simulink model "zynqRadioHWSWLTEDetectorAD9361AD9364SL"  (R2016a)
settings: Solver=FixedStepDiscrete  SolverMode=SingleTasking  StartTime=0.0  StopTime=inf  RelTol=1e-3
InitFcn:
  | % Load LTE detector initialization parameters
  | simParams = hdlcoder_lteofdm_modDetectref_init;
  | simParams = hdlcoder_lteofdm_modDetecthdl_init(simParams);
  | 
  | % Modify PSS detection threshold gain for modified
  | % front-end filter
  | simParams.thresholdGain = 16;
  | 
  | % Load LTE TX waveforms
  | load('zynqRadioLTETransmitData');
libraries: simulink x26, hdlsllib x18, dspsigops x3, dspxfrm3 x1, dspmlti4 x1, dspmathops x1, dspsrcs4 x1
(part 2 of 2)

== system zynqRadioHWSWLTEDetectorAD9361AD9364SL/HDL_LTE/PSS_Detection/Cross_Correlation/Magnitude_Squared_0 ==
  dataIn : Inport
  Add : Sum  OutDataTypeStr=Inherit: Same as accumulator
  Complex to Real-Imag : ComplexToRealImag
  Delay1 : Delay  InitialCondition=0
  Delay2 : Delay  InitialCondition=0
  Delay3 : Delay  DelayLength=1  InitialCondition=0
  Delay4 : Delay  InitialCondition=0
  Product4 : Product
  Product5 : Product
  Magnitude^2 : Outport
  wires:
  Delay4/1 -> Magnitude^2/1
  Delay2/1 -> Add/2
  Delay1/1 -> Add/1
  Delay3/1 -> Complex to Real-Imag/1
  dataIn/1 -> Delay3/1
  Product4/1 -> Delay1/1
  Complex to Real-Imag/2 -> Product5/1, Product5/2
  Complex to Real-Imag/1 -> Product4/1, Product4/2
  Add/1 -> Delay4/1
  Product5/1 -> Delay2/1

== system zynqRadioHWSWLTEDetectorAD9361AD9364SL/HDL_LTE/PSS_Detection/Cross_Correlation/Magnitude_Squared_1 ==
  dataIn : Inport
  Add : Sum  OutDataTypeStr=Inherit: Same as accumulator
  Complex to Real-Imag : ComplexToRealImag
  Delay1 : Delay  InitialCondition=0
  Delay2 : Delay  InitialCondition=0
  Delay3 : Delay  DelayLength=1  InitialCondition=0
  Delay4 : Delay  InitialCondition=0
  Product4 : Product
  Product5 : Product
  Magnitude^2 : Outport
  wires:
  Delay4/1 -> Magnitude^2/1
  Delay2/1 -> Add/2
  Delay1/1 -> Add/1
  Delay3/1 -> Complex to Real-Imag/1
  dataIn/1 -> Delay3/1
  Product4/1 -> Delay1/1
  Complex to Real-Imag/2 -> Product5/1, Product5/2
  Complex to Real-Imag/1 -> Product4/1, Product4/2
  Add/1 -> Delay4/1
  Product5/1 -> Delay2/1

== system zynqRadioHWSWLTEDetectorAD9361AD9364SL/HDL_LTE/PSS_Detection/Cross_Correlation/Magnitude_Squared_2 ==
  dataIn : Inport
  Add : Sum  OutDataTypeStr=Inherit: Same as accumulator
  Complex to Real-Imag : ComplexToRealImag
  Delay1 : Delay  InitialCondition=0
  Delay2 : Delay  InitialCondition=0
  Delay3 : Delay  DelayLength=1  InitialCondition=0
  Delay4 : Delay  InitialCondition=0
  Product4 : Product
  Product5 : Product
  Magnitude^2 : Outport
  wires:
  Delay4/1 -> Magnitude^2/1
  Delay2/1 -> Add/2
  Delay1/1 -> Add/1
  Delay3/1 -> Complex to Real-Imag/1
  dataIn/1 -> Delay3/1
  Product4/1 -> Delay1/1
  Complex to Real-Imag/2 -> Product5/1, Product5/2
  Complex to Real-Imag/1 -> Product4/1, Product4/2
  Add/1 -> Delay4/1
  Product5/1 -> Delay2/1

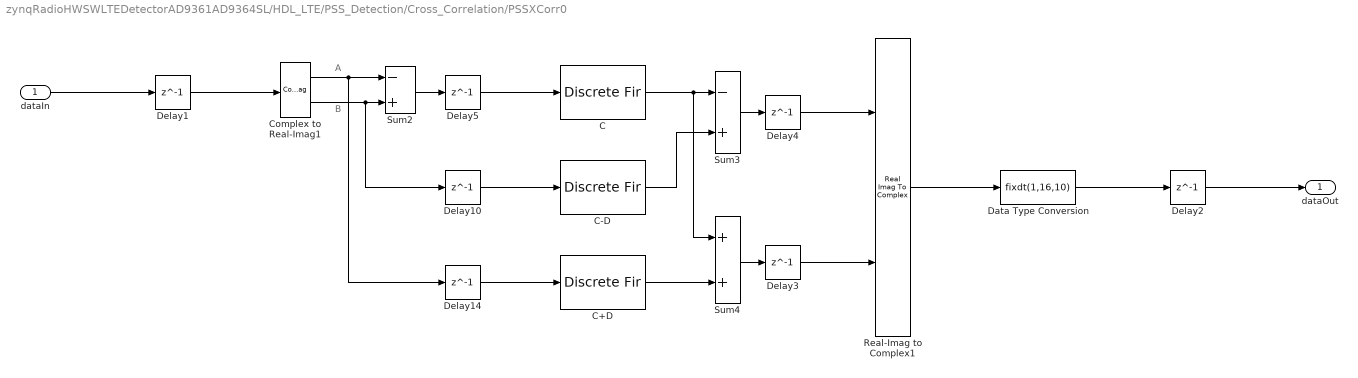
== system zynqRadioHWSWLTEDetectorAD9361AD9364SL/HDL_LTE/PSS_Detection/Cross_Correlation/PSSXCorr0 ==
  note: B
  note: A
  dataIn : Inport
  C : DiscreteFir  Coefficients=real(simParams.PSS(:,PSSIdx+1)')  CoefDataTypeStr=fixdt(1,18)
  C+D : DiscreteFir  Coefficients=real(simParams.PSS(:,PSSIdx+1)') + imag(simParams.PSS(:,PSSIdx+1)')  CoefDataTypeStr=fixdt(1,18)
  C-D : DiscreteFir  Coefficients=real(simParams.PSS(:,PSSIdx+1)') - imag(simParams.PSS(:,PSSIdx+1)')  CoefDataTypeStr=fixdt(1,18)
  Complex to Real-Imag1 : ComplexToRealImag
  Data Type Conversion : DataTypeConversion  OutDataTypeStr=fixdt(1,16,10)  RndMeth=Round
  Delay{1..5,10,14} (7 alike) : Delay  DelayLength=1  InitialCondition=0
  Real-Imag to Complex1 : RealImagToComplex
  Sum2 : Sum  Inputs=-+
  Sum3 : Sum  Inputs=-+
  Sum4 : Sum
  dataOut : Outport
  wires:
  dataIn/1 -> Delay1/1
  Real-Imag to Complex1/1 -> Data Type Conversion/1
  Sum2/1 -> Delay5/1
  Complex to Real-Imag1/1 -> Delay14/1, Sum2/1
  Complex to Real-Imag1/2 -> Delay10/1, Sum2/2
  C/1 -> Sum4/1, Sum3/1
  C-D/1 -> Sum3/2
  C+D/1 -> Sum4/2
  Sum3/1 -> Delay4/1
  Sum4/1 -> Delay3/1
  Delay1/1 -> Complex to Real-Imag1/1
  Delay2/1 -> dataOut/1
  Delay3/1 -> Real-Imag to Complex1/2
  Delay4/1 -> Real-Imag to Complex1/1
  Delay5/1 -> C/1
  Delay10/1 -> C-D/1
  Delay14/1 -> C+D/1
  Data Type Conversion/1 -> Delay2/1

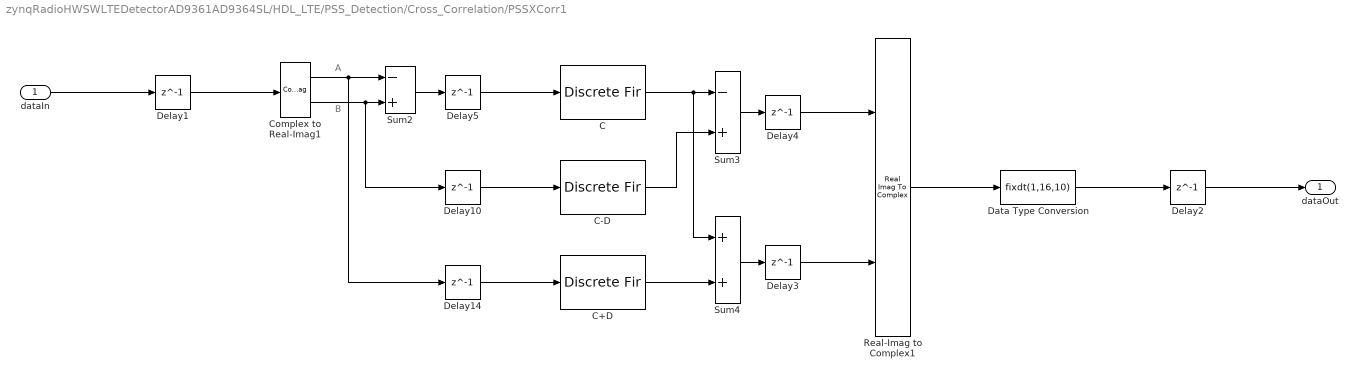
== system zynqRadioHWSWLTEDetectorAD9361AD9364SL/HDL_LTE/PSS_Detection/Cross_Correlation/PSSXCorr1 ==
  note: B
  note: A
  dataIn : Inport
  C : DiscreteFir  Coefficients=real(simParams.PSS(:,PSSIdx+1)')  CoefDataTypeStr=fixdt(1,18)
  C+D : DiscreteFir  Coefficients=real(simParams.PSS(:,PSSIdx+1)') + imag(simParams.PSS(:,PSSIdx+1)')  CoefDataTypeStr=fixdt(1,18)
  C-D : DiscreteFir  Coefficients=real(simParams.PSS(:,PSSIdx+1)') - imag(simParams.PSS(:,PSSIdx+1)')  CoefDataTypeStr=fixdt(1,18)
  Complex to Real-Imag1 : ComplexToRealImag
  Data Type Conversion : DataTypeConversion  OutDataTypeStr=fixdt(1,16,10)  RndMeth=Round
  Delay{1..5,10,14} (7 alike) : Delay  DelayLength=1  InitialCondition=0
  Real-Imag to Complex1 : RealImagToComplex
  Sum2 : Sum  Inputs=-+
  Sum3 : Sum  Inputs=-+
  Sum4 : Sum
  dataOut : Outport
  wires:
  dataIn/1 -> Delay1/1
  Real-Imag to Complex1/1 -> Data Type Conversion/1
  Sum2/1 -> Delay5/1
  Complex to Real-Imag1/1 -> Delay14/1, Sum2/1
  Complex to Real-Imag1/2 -> Delay10/1, Sum2/2
  C/1 -> Sum4/1, Sum3/1
  C-D/1 -> Sum3/2
  C+D/1 -> Sum4/2
  Sum3/1 -> Delay4/1
  Sum4/1 -> Delay3/1
  Delay1/1 -> Complex to Real-Imag1/1
  Delay2/1 -> dataOut/1
  Delay3/1 -> Real-Imag to Complex1/2
  Delay4/1 -> Real-Imag to Complex1/1
  Delay5/1 -> C/1
  Delay10/1 -> C-D/1
  Delay14/1 -> C+D/1
  Data Type Conversion/1 -> Delay2/1

== system zynqRadioHWSWLTEDetectorAD9361AD9364SL/HDL_LTE/PSS_Detection/Cross_Correlation/PSSXCorr2 ==
  note: B
  note: A
  dataIn : Inport
  C : DiscreteFir  Coefficients=real(simParams.PSS(:,PSSIdx+1)')  CoefDataTypeStr=fixdt(1,18)
  C+D : DiscreteFir  Coefficients=real(simParams.PSS(:,PSSIdx+1)') + imag(simParams.PSS(:,PSSIdx+1)')  CoefDataTypeStr=fixdt(1,18)
  C-D : DiscreteFir  Coefficients=real(simParams.PSS(:,PSSIdx+1)') - imag(simParams.PSS(:,PSSIdx+1)')  CoefDataTypeStr=fixdt(1,18)
  Complex to Real-Imag1 : ComplexToRealImag
  Data Type Conversion : DataTypeConversion  OutDataTypeStr=fixdt(1,16,10)  RndMeth=Round
  Delay{1..5,10,14} (7 alike) : Delay  DelayLength=1  InitialCondition=0
  Real-Imag to Complex1 : RealImagToComplex
  Sum2 : Sum  Inputs=-+
  Sum3 : Sum  Inputs=-+
  Sum4 : Sum
  dataOut : Outport
  wires:
  dataIn/1 -> Delay1/1
  Real-Imag to Complex1/1 -> Data Type Conversion/1
  Sum2/1 -> Delay5/1
  Complex to Real-Imag1/1 -> Delay14/1, Sum2/1
  Complex to Real-Imag1/2 -> Delay10/1, Sum2/2
  C/1 -> Sum4/1, Sum3/1
  C-D/1 -> Sum3/2
  C+D/1 -> Sum4/2
  Sum3/1 -> Delay4/1
  Sum4/1 -> Delay3/1
  Delay1/1 -> Complex to Real-Imag1/1
  Delay2/1 -> dataOut/1
  Delay3/1 -> Real-Imag to Complex1/2
  Delay4/1 -> Real-Imag to Complex1/1
  Delay5/1 -> C/1
  Delay10/1 -> C-D/1
  Delay14/1 -> C+D/1
  Data Type Conversion/1 -> Delay2/1

== system zynqRadioHWSWLTEDetectorAD9361AD9364SL/HDL_LTE/PSS_Detection/Peak_Detection/Local_Search_PSS0 ==
  note: Generate 10 sample enable signal
  Enb : Inport
  dataIn : Inport  Port=2
  indexIn : Inport  Port=3
  Add : Sum  AccumDataTypeStr=fixdt(0,15,0)
  Constant1 : Constant  Value=0  VectorParams1D=off  OutDataTypeStr=fixdt(0,22,20)  SampleTime=simParams.TsRx
  Constant2 : Constant  Value=11  VectorParams1D=off  OutDataTypeStr=fixdt(0,4,0)  SampleTime=simParams.TsRx
  Delay1 : Delay  DelayLength=11  InitialCondition=0
  Delay2 : Delay  DelayLength=1  InitialCondition=0
  Delay21 : Delay  DelayLength=1  InitialCondition=0  InputProcessing=Columns as channels (frame based)
  Delay3 : Delay  DelayLength=1  InitialCondition=0  InputProcessing=Columns as channels (frame based)
  HDL Counter : hdlsllib/HDL Operations/HDL Counter  CountType=Count limited  CountInit=1  CountStep=1  CountMax=11  CountFromType=Initial value  CountFrom=1  CountResetPort=off  CountLoadPort=off  CountEnbPort=on  CountDirPort=off  CountDataType=Unsigned  CountWordLen=4  CountFracLen=0  CountSampTime=1
  Logical Operator2 : Logic  Operator=OR  AllPortsSameDT=off  OutDataTypeStr=boolean
  Relational Operator1 : RelationalOperator  Operator=<  OutDataTypeStr=boolean
  Relational Operator2 : RelationalOperator  Operator=>  OutDataTypeStr=boolean
  Switch1 : Switch  Criteria=u2 ~= 0  Threshold=384
  maximum : Subsystem
  MaxIdx : Outport
  MaxVal : Outport  Port=2
  wires:
  Enb/1 -> Logical Operator2/1
  maximum/1(MaxVal) -> Delay21/1
  dataIn/1 -> Delay2/1
  maximum/2(MaxIdx) -> Relational Operator2/1, Add/1
  Add/1 -> Delay3/1
  Relational Operator2/1 -> Switch1/2
  indexIn/1 -> Delay1/1
  Constant1/1 -> Switch1/3, Relational Operator2/2
  Switch1/1 -> Add/2
  Delay1/1 -> Switch1/1
  Constant2/1 -> Relational Operator1/2
  Logical Operator2/1 -> HDL Counter/1
  Relational Operator1/1 -> maximum/2(Enb), Logical Operator2/2
  Delay2/1 -> maximum/1(dataIn)
  Delay21/1 -> MaxVal/1
  Delay3/1 -> MaxIdx/1
  HDL Counter/1 -> Relational Operator1/1

== system zynqRadioHWSWLTEDetectorAD9361AD9364SL/HDL_LTE/PSS_Detection/Peak_Detection/Local_Search_PSS1 ==
  note: Generate 10 sample enable signal
  Enb : Inport
  dataIn : Inport  Port=2
  indexIn : Inport  Port=3
  Add : Sum  AccumDataTypeStr=fixdt(0,15,0)
  Constant1 : Constant  Value=0  VectorParams1D=off  OutDataTypeStr=fixdt(0,22,20)  SampleTime=simParams.TsRx
  Constant2 : Constant  Value=11  VectorParams1D=off  OutDataTypeStr=fixdt(0,4,0)  SampleTime=simParams.TsRx
  Delay1 : Delay  DelayLength=11  InitialCondition=0
  Delay2 : Delay  DelayLength=1  InitialCondition=0
  Delay21 : Delay  DelayLength=1  InitialCondition=0  InputProcessing=Columns as channels (frame based)
  Delay3 : Delay  DelayLength=1  InitialCondition=0  InputProcessing=Columns as channels (frame based)
  HDL Counter : hdlsllib/HDL Operations/HDL Counter  CountType=Count limited  CountInit=1  CountStep=1  CountMax=11  CountFromType=Initial value  CountFrom=1  CountResetPort=off  CountLoadPort=off  CountEnbPort=on  CountDirPort=off  CountDataType=Unsigned  CountWordLen=4  CountFracLen=0  CountSampTime=1
  Logical Operator2 : Logic  Operator=OR  AllPortsSameDT=off  OutDataTypeStr=boolean
  Relational Operator1 : RelationalOperator  Operator=<  OutDataTypeStr=boolean
  Relational Operator2 : RelationalOperator  Operator=>  OutDataTypeStr=boolean
  Switch1 : Switch  Criteria=u2 ~= 0  Threshold=384
  maximum : Subsystem
  MaxIdx : Outport
  MaxVal : Outport  Port=2
  wires:
  HDL Counter/1 -> Relational Operator1/1
  Delay3/1 -> MaxIdx/1
  Delay21/1 -> MaxVal/1
  Delay2/1 -> maximum/1(dataIn)
  Relational Operator1/1 -> Logical Operator2/2, maximum/2(Enb)
  Logical Operator2/1 -> HDL Counter/1
  Constant2/1 -> Relational Operator1/2
  Delay1/1 -> Switch1/1
  Switch1/1 -> Add/2
  Constant1/1 -> Relational Operator2/2, Switch1/3
  indexIn/1 -> Delay1/1
  Relational Operator2/1 -> Switch1/2
  Add/1 -> Delay3/1
  maximum/2(MaxIdx) -> Add/1, Relational Operator2/1
  dataIn/1 -> Delay2/1
  maximum/1(MaxVal) -> Delay21/1
  Enb/1 -> Logical Operator2/1

== system zynqRadioHWSWLTEDetectorAD9361AD9364SL/HDL_LTE/PSS_Detection/Peak_Detection/Local_Search_PSS2 ==
  note: Generate 10 sample enable signal
  Enb : Inport
  dataIn : Inport  Port=2
  indexIn : Inport  Port=3
  Add : Sum  AccumDataTypeStr=fixdt(0,15,0)
  Constant1 : Constant  Value=0  VectorParams1D=off  OutDataTypeStr=fixdt(0,22,20)  SampleTime=simParams.TsRx
  Constant2 : Constant  Value=11  VectorParams1D=off  OutDataTypeStr=fixdt(0,4,0)  SampleTime=simParams.TsRx
  Delay1 : Delay  DelayLength=11  InitialCondition=0
  Delay2 : Delay  DelayLength=1  InitialCondition=0
  Delay21 : Delay  DelayLength=1  InitialCondition=0  InputProcessing=Columns as channels (frame based)
  Delay3 : Delay  DelayLength=1  InitialCondition=0  InputProcessing=Columns as channels (frame based)
  HDL Counter : hdlsllib/HDL Operations/HDL Counter  CountType=Count limited  CountInit=1  CountStep=1  CountMax=11  CountFromType=Initial value  CountFrom=1  CountResetPort=off  CountLoadPort=off  CountEnbPort=on  CountDirPort=off  CountDataType=Unsigned  CountWordLen=4  CountFracLen=0  CountSampTime=1
  Logical Operator2 : Logic  Operator=OR  AllPortsSameDT=off  OutDataTypeStr=boolean
  Relational Operator1 : RelationalOperator  Operator=<  OutDataTypeStr=boolean
  Relational Operator2 : RelationalOperator  Operator=>  OutDataTypeStr=boolean
  Switch1 : Switch  Criteria=u2 ~= 0  Threshold=384
  maximum : Subsystem
  MaxIdx : Outport
  MaxVal : Outport  Port=2
  wires:
  Enb/1 -> Logical Operator2/1
  maximum/1(MaxVal) -> Delay21/1
  dataIn/1 -> Delay2/1
  maximum/2(MaxIdx) -> Relational Operator2/1, Add/1
  Add/1 -> Delay3/1
  Relational Operator2/1 -> Switch1/2
  indexIn/1 -> Delay1/1
  Constant1/1 -> Switch1/3, Relational Operator2/2
  Switch1/1 -> Add/2
  Delay1/1 -> Switch1/1
  Constant2/1 -> Relational Operator1/2
  Logical Operator2/1 -> HDL Counter/1
  Relational Operator1/1 -> maximum/2(Enb), Logical Operator2/2
  Delay2/1 -> maximum/1(dataIn)
  Delay21/1 -> MaxVal/1
  Delay3/1 -> MaxIdx/1
  HDL Counter/1 -> Relational Operator1/1

== system zynqRadioHWSWLTEDetectorAD9361AD9364SL/HDL_LTE/SSS_Detection/SSS_Dot_Product/Delay Reset ==
  note: Enable
  u : Inport
  E : Inport  Port=2
  R : Inport  Port=3
  Enable : Switch  Criteria=u2 > Threshold  OutDataTypeStr=Inherit: Inherit via back propagation  ZeroCross=off
  Reset Delay : Subsystem
  y : Outport
  wires:
  R/1 -> Reset Delay/2(R1)
  Enable/1 -> Reset Delay/1(u1)
  u/1 -> Enable/1
  Reset Delay/1(Out1) -> y/1, Enable/3
  E/1 -> Enable/2

== system zynqRadioHWSWLTEDetectorAD9361AD9364SL/HDL_LTE/SSS_Detection/SSS_Dot_Product/Magnitude Squared 0 ==
  dataIn : Inport
  Add : Sum  OutDataTypeStr=Inherit: Same as first input
  Complex to Real-Imag : ComplexToRealImag
  Delay1 : Delay  InitialCondition=0
  Delay2 : Delay  InitialCondition=0
  Delay3 : Delay  DelayLength=1  InitialCondition=0
  Delay4 : Delay  InitialCondition=0
  Product4 : Product
  Product5 : Product
  Magnitude^2 : Outport
  wires:
  Delay4/1 -> Magnitude^2/1
  Delay2/1 -> Add/2
  Delay1/1 -> Add/1
  Delay3/1 -> Complex to Real-Imag/1
  dataIn/1 -> Delay3/1
  Product4/1 -> Delay1/1
  Complex to Real-Imag/2 -> Product5/1, Product5/2
  Complex to Real-Imag/1 -> Product4/1, Product4/2
  Add/1 -> Delay4/1
  Product5/1 -> Delay2/1

== system zynqRadioHWSWLTEDetectorAD9361AD9364SL/HDL_LTE/SSS_Detection/Sample_and_Store/LUT Toggle Counters ==
  In1 : Inport
  Compare To Constant4 : simulink/Logic and Bit Operations/Compare To Constant  relop===  const=255  OutDataTypeStr=boolean
  Compare To Constant5 : simulink/Logic and Bit Operations/Compare To Constant  relop=<  const=128  OutDataTypeStr=boolean
  Index SubFrame 0 : hdlsllib/HDL Operations/HDL Counter  CountType=Count limited  CountInit=0  CountStep=1  CountMax=167  CountFromType=Initial value  CountFrom=0  CountResetPort=off  CountLoadPort=off  CountEnbPort=on  CountDirPort=off  CountDataType=Unsigned  CountWordLen=ceil(log2(167))  CountFracLen=0  CountSampTime=1
  Index SubFrame 5 : hdlsllib/HDL Operations/HDL Counter  CountType=Count limited  CountInit=168  CountStep=1  CountMax=335  CountFromType=Initial value  CountFrom=168  CountResetPort=off  CountLoadPort=off  CountEnbPort=on  CountDirPort=off  CountDataType=Unsigned  CountWordLen=ceil(log2(335))  CountFracLen=0  CountSampTime=1
  Sample Counter1 : hdlsllib/HDL Operations/HDL Counter  CountType=Count limited  CountInit=0  CountStep=1  CountMax=255  CountFromType=Initial value  CountFrom=0  CountResetPort=off  CountLoadPort=off  CountEnbPort=on  CountDirPort=off  CountDataType=Unsigned  CountWordLen=ceil(log2(255))  CountFracLen=0  CountSampTime=1
  Switch4 : Switch  Criteria=u2 ~= 0
  Out1 : Outport
  Out2 : Outport  Port=2
  wires:
  Index SubFrame 5/1 -> Switch4/3
  Compare To Constant4/1 -> Index SubFrame 5/1, Index SubFrame 0/1
  Sample Counter1/1 -> Compare To Constant5/1, Compare To Constant4/1
  Compare To Constant5/1 -> Switch4/2
  Index SubFrame 0/1 -> Out2/1, Switch4/1
  In1/1 -> Sample Counter1/1
  Switch4/1 -> Out1/1

== system zynqRadioHWSWLTEDetectorAD9361AD9364SL/HDL_LTE/PSS_Detection/Peak_Detection/Local_Search_PSS0/maximum ==
  note: After 10 clock cycles, output
      | maximum value and corresponding
      | index value
  note: Hold index value (out of 10)
      | for current maximum value
  note: Count to 10
  note: Check for new maximum value
  dataIn : Inport
  Enb : Inport  Port=2
  Constant : Constant  Value=10  VectorParams1D=off  OutDataTypeStr=fixdt(0,4,0)  SampleTime=simParams.TsRx
  Constant1 : Constant  Value=0  VectorParams1D=off  OutDataTypeStr=fixdt(0,22,20)  SampleTime=simParams.TsRx
  Delay Reset : Subsystem
  Delay Reset2 : Subsystem
  HDL Counter : hdlsllib/HDL Operations/HDL Counter  CountType=Count limited  CountInit=1  CountStep=1  CountMax=10  CountFromType=Initial value  CountFrom=1  CountResetPort=on  CountLoadPort=off  CountEnbPort=on  CountDirPort=off  CountDataType=Unsigned  CountWordLen=4  CountFracLen=0  CountSampTime=1
  Logical Operator1 : Logic  Operator=NOT  IconShape=distinctive  AllPortsSameDT=off  OutDataTypeStr=boolean
  Relational Operator1 : RelationalOperator  Operator=>  OutDataTypeStr=boolean
  Relational Operator2 : RelationalOperator  Operator===  OutDataTypeStr=boolean
  Switch : Switch  Criteria=u2 > Threshold
  Switch1 : Switch  Criteria=u2 > Threshold
  MaxVal : Outport  InitialOutput=0
  MaxIdx : Outport  Port=2  InitialOutput=0
  wires:
  Relational Operator1/1 -> Delay Reset2/2(E), Delay Reset/2(E)
  Delay Reset/1(y) -> Switch/1, Relational Operator1/2
  Enb/1 -> Logical Operator1/1, HDL Counter/2
  dataIn/1 -> Delay Reset/1(u), Relational Operator1/1
  Constant/1 -> Relational Operator2/2
  Switch/1 -> MaxVal/1
  Relational Operator2/1 -> Switch/2, Switch1/2
  Constant1/1 -> Switch/3, Switch1/3
  Switch1/1 -> MaxIdx/1
  Delay Reset2/1(y) -> Switch1/1
  Logical Operator1/1 -> HDL Counter/1, Delay Reset2/3(R), Delay Reset/3(R)
  HDL Counter/1 -> Delay Reset2/1(u), Relational Operator2/1

== system zynqRadioHWSWLTEDetectorAD9361AD9364SL/HDL_LTE/PSS_Detection/Peak_Detection/Local_Search_PSS1/maximum ==
  note: Check for new maximum value
  note: Count to 10
  note: Hold index value (out of 10)
      | for current maximum value
  note: After 10 clock cycles, output
      | maximum value and corresponding
      | index value
  dataIn : Inport
  Enb : Inport  Port=2
  Constant : Constant  Value=10  VectorParams1D=off  OutDataTypeStr=fixdt(0,4,0)  SampleTime=simParams.TsRx
  Constant1 : Constant  Value=0  VectorParams1D=off  OutDataTypeStr=fixdt(0,22,20)  SampleTime=simParams.TsRx
  Delay Reset : Subsystem
  Delay Reset2 : Subsystem
  HDL Counter : hdlsllib/HDL Operations/HDL Counter  CountType=Count limited  CountInit=1  CountStep=1  CountMax=10  CountFromType=Initial value  CountFrom=1  CountResetPort=on  CountLoadPort=off  CountEnbPort=on  CountDirPort=off  CountDataType=Unsigned  CountWordLen=4  CountFracLen=0  CountSampTime=1
  Logical Operator1 : Logic  Operator=NOT  IconShape=distinctive  AllPortsSameDT=off  OutDataTypeStr=boolean
  Relational Operator1 : RelationalOperator  Operator=>  OutDataTypeStr=boolean
  Relational Operator2 : RelationalOperator  Operator===  OutDataTypeStr=boolean
  Switch : Switch  Criteria=u2 > Threshold
  Switch1 : Switch  Criteria=u2 > Threshold
  MaxVal : Outport  InitialOutput=0
  MaxIdx : Outport  Port=2  InitialOutput=0
  wires:
  HDL Counter/1 -> Relational Operator2/1, Delay Reset2/1(u)
  Logical Operator1/1 -> Delay Reset/3(R), Delay Reset2/3(R), HDL Counter/1
  Delay Reset2/1(y) -> Switch1/1
  Switch1/1 -> MaxIdx/1
  Constant1/1 -> Switch1/3, Switch/3
  Relational Operator2/1 -> Switch1/2, Switch/2
  Switch/1 -> MaxVal/1
  Constant/1 -> Relational Operator2/2
  dataIn/1 -> Relational Operator1/1, Delay Reset/1(u)
  Enb/1 -> HDL Counter/2, Logical Operator1/1
  Delay Reset/1(y) -> Relational Operator1/2, Switch/1
  Relational Operator1/1 -> Delay Reset/2(E), Delay Reset2/2(E)

== system zynqRadioHWSWLTEDetectorAD9361AD9364SL/HDL_LTE/PSS_Detection/Peak_Detection/Local_Search_PSS2/maximum ==
  note: After 10 clock cycles, output
      | maximum value and corresponding
      | index value
  note: Hold index value (out of 10)
      | for current maximum value
  note: Count to 10
  note: Check for new maximum value
  dataIn : Inport
  Enb : Inport  Port=2
  Constant : Constant  Value=10  VectorParams1D=off  OutDataTypeStr=fixdt(0,4,0)  SampleTime=simParams.TsRx
  Constant1 : Constant  Value=0  VectorParams1D=off  OutDataTypeStr=fixdt(0,22,20)  SampleTime=simParams.TsRx
  Delay Reset : Subsystem
  Delay Reset2 : Subsystem
  HDL Counter : hdlsllib/HDL Operations/HDL Counter  CountType=Count limited  CountInit=1  CountStep=1  CountMax=10  CountFromType=Initial value  CountFrom=1  CountResetPort=on  CountLoadPort=off  CountEnbPort=on  CountDirPort=off  CountDataType=Unsigned  CountWordLen=4  CountFracLen=0  CountSampTime=1
  Logical Operator1 : Logic  Operator=NOT  IconShape=distinctive  AllPortsSameDT=off  OutDataTypeStr=boolean
  Relational Operator1 : RelationalOperator  Operator=>  OutDataTypeStr=boolean
  Relational Operator2 : RelationalOperator  Operator===  OutDataTypeStr=boolean
  Switch : Switch  Criteria=u2 > Threshold
  Switch1 : Switch  Criteria=u2 > Threshold
  MaxVal : Outport  InitialOutput=0
  MaxIdx : Outport  Port=2  InitialOutput=0
  wires:
  Relational Operator1/1 -> Delay Reset2/2(E), Delay Reset/2(E)
  Delay Reset/1(y) -> Switch/1, Relational Operator1/2
  Enb/1 -> Logical Operator1/1, HDL Counter/2
  dataIn/1 -> Delay Reset/1(u), Relational Operator1/1
  Constant/1 -> Relational Operator2/2
  Switch/1 -> MaxVal/1
  Relational Operator2/1 -> Switch/2, Switch1/2
  Constant1/1 -> Switch/3, Switch1/3
  Switch1/1 -> MaxIdx/1
  Delay Reset2/1(y) -> Switch1/1
  Logical Operator1/1 -> HDL Counter/1, Delay Reset2/3(R), Delay Reset/3(R)
  HDL Counter/1 -> Delay Reset2/1(u), Relational Operator2/1

== system zynqRadioHWSWLTEDetectorAD9361AD9364SL/HDL_LTE/SSS_Detection/SSS_Dot_Product/Delay Reset/Reset Delay ==
  note: Reset
  u1 : Inport
  R1 : Inport  Port=2
  FixPt Constant : Constant  DisableCoverage=on  Value=0  OutDataTypeStr=uint8  SampleTime=simParams.TsRx
  FixPt Logical Operator : Logic  DisableCoverage=on  Operator=OR  AllPortsSameDT=off  OutDataTypeStr=fixdt(0, 8)
  FixPt Unit Delay1 : UnitDelay  DisableCoverage=on  SampleTime=-1  HasFrameUpgradeWarning=off
  FixPt Unit Delay2 : UnitDelay  DisableCoverage=on  InitialCondition=1  SampleTime=-1
  Init : Switch  Criteria=u2 > Threshold  OutDataTypeStr=Inherit: Inherit via back propagation  ZeroCross=off
  Initial Condition : Constant  DisableCoverage=on  Value=complex(0)  OutDataTypeStr=Inherit: Inherit via back propagation  SampleTime=simParams.TsRx
  Reset : Switch  Criteria=u2 > Threshold  OutDataTypeStr=Inherit: Inherit via back propagation  ZeroCross=off
  Out1 : Outport
  wires:
  Reset/1 -> FixPt Unit Delay1/1  "Xnew"
  Init/1 -> Out1/1
  R1/1 -> Reset/2, FixPt Logical Operator/1
  FixPt Logical Operator/1 -> Init/2
  FixPt Unit Delay2/1 -> FixPt Logical Operator/2
  FixPt Constant/1 -> FixPt Unit Delay2/1
  Initial Condition/1 -> Reset/1, Init/1  "Initial Value"
  FixPt Unit Delay1/1 -> Init/3  "Xold"
  u1/1 -> Reset/3

== system zynqRadioHWSWLTEDetectorAD9361AD9364SL/HDL_LTE/PSS_Detection/Peak_Detection/Local_Search_PSS0/maximum/Delay Reset ==
  note: Enable
  u : Inport
  E : Inport  Port=2
  R : Inport  Port=3
  Enable : Switch  Criteria=u2 > Threshold  OutDataTypeStr=Inherit: Inherit via back propagation  ZeroCross=off
  Reset Delay : Subsystem
  y : Outport
  wires:
  E/1 -> Enable/2
  Reset Delay/1(Out1) -> Enable/3, y/1
  u/1 -> Enable/1
  Enable/1 -> Reset Delay/1(u1)
  R/1 -> Reset Delay/2(R1)

== system zynqRadioHWSWLTEDetectorAD9361AD9364SL/HDL_LTE/PSS_Detection/Peak_Detection/Local_Search_PSS0/maximum/Delay Reset2 ==
  note: Enable
  u : Inport
  E : Inport  Port=2
  R : Inport  Port=3
  Enable : Switch  Criteria=u2 > Threshold  OutDataTypeStr=Inherit: Inherit via back propagation  ZeroCross=off
  Reset Delay : Subsystem
  y : Outport
  wires:
  E/1 -> Enable/2
  Reset Delay/1(Out1) -> Enable/3, y/1
  u/1 -> Enable/1
  Enable/1 -> Reset Delay/1(u1)
  R/1 -> Reset Delay/2(R1)

== system zynqRadioHWSWLTEDetectorAD9361AD9364SL/HDL_LTE/PSS_Detection/Peak_Detection/Local_Search_PSS1/maximum/Delay Reset ==
  note: Enable
  u : Inport
  E : Inport  Port=2
  R : Inport  Port=3
  Enable : Switch  Criteria=u2 > Threshold  OutDataTypeStr=Inherit: Inherit via back propagation  ZeroCross=off
  Reset Delay : Subsystem
  y : Outport
  wires:
  R/1 -> Reset Delay/2(R1)
  Enable/1 -> Reset Delay/1(u1)
  u/1 -> Enable/1
  Reset Delay/1(Out1) -> y/1, Enable/3
  E/1 -> Enable/2

== system zynqRadioHWSWLTEDetectorAD9361AD9364SL/HDL_LTE/PSS_Detection/Peak_Detection/Local_Search_PSS1/maximum/Delay Reset2 ==
  note: Enable
  u : Inport
  E : Inport  Port=2
  R : Inport  Port=3
  Enable : Switch  Criteria=u2 > Threshold  OutDataTypeStr=Inherit: Inherit via back propagation  ZeroCross=off
  Reset Delay : Subsystem
  y : Outport
  wires:
  R/1 -> Reset Delay/2(R1)
  Enable/1 -> Reset Delay/1(u1)
  u/1 -> Enable/1
  Reset Delay/1(Out1) -> y/1, Enable/3
  E/1 -> Enable/2

== system zynqRadioHWSWLTEDetectorAD9361AD9364SL/HDL_LTE/PSS_Detection/Peak_Detection/Local_Search_PSS2/maximum/Delay Reset ==
  note: Enable
  u : Inport
  E : Inport  Port=2
  R : Inport  Port=3
  Enable : Switch  Criteria=u2 > Threshold  OutDataTypeStr=Inherit: Inherit via back propagation  ZeroCross=off
  Reset Delay : Subsystem
  y : Outport
  wires:
  E/1 -> Enable/2
  Reset Delay/1(Out1) -> Enable/3, y/1
  u/1 -> Enable/1
  Enable/1 -> Reset Delay/1(u1)
  R/1 -> Reset Delay/2(R1)

== system zynqRadioHWSWLTEDetectorAD9361AD9364SL/HDL_LTE/PSS_Detection/Peak_Detection/Local_Search_PSS2/maximum/Delay Reset2 ==
  note: Enable
  u : Inport
  E : Inport  Port=2
  R : Inport  Port=3
  Enable : Switch  Criteria=u2 > Threshold  OutDataTypeStr=Inherit: Inherit via back propagation  ZeroCross=off
  Reset Delay : Subsystem
  y : Outport
  wires:
  E/1 -> Enable/2
  Reset Delay/1(Out1) -> Enable/3, y/1
  u/1 -> Enable/1
  Enable/1 -> Reset Delay/1(u1)
  R/1 -> Reset Delay/2(R1)

== system zynqRadioHWSWLTEDetectorAD9361AD9364SL/HDL_LTE/PSS_Detection/Peak_Detection/Local_Search_PSS0/maximum/Delay Reset/Reset Delay ==
  note: Reset
  u1 : Inport
  R1 : Inport  Port=2
  FixPt Constant : Constant  DisableCoverage=on  Value=0  OutDataTypeStr=fixdt(0,8,0)  SampleTime=simParams.TsRx
  FixPt Logical Operator : Logic  DisableCoverage=on  Operator=OR  AllPortsSameDT=off  OutDataTypeStr=fixdt(0, 8)
  FixPt Unit Delay1 : UnitDelay  DisableCoverage=on  SampleTime=-1  HasFrameUpgradeWarning=off
  FixPt Unit Delay2 : UnitDelay  DisableCoverage=on  InitialCondition=1  SampleTime=-1
  Init : Switch  Criteria=u2 > Threshold  OutDataTypeStr=Inherit: Inherit via back propagation  ZeroCross=off
  Initial Condition : Constant  DisableCoverage=on  Value=0  OutDataTypeStr=Inherit: Inherit via back propagation  SampleTime=simParams.TsRx
  Reset : Switch  Criteria=u2 > Threshold  OutDataTypeStr=Inherit: Inherit via back propagation  ZeroCross=off
  Out1 : Outport
  wires:
  u1/1 -> Reset/3
  FixPt Unit Delay1/1 -> Init/3  "Xold"
  Initial Condition/1 -> Init/1, Reset/1  "Initial Value"
  FixPt Constant/1 -> FixPt Unit Delay2/1
  FixPt Unit Delay2/1 -> FixPt Logical Operator/2
  FixPt Logical Operator/1 -> Init/2
  R1/1 -> FixPt Logical Operator/1, Reset/2
  Init/1 -> Out1/1
  Reset/1 -> FixPt Unit Delay1/1  "Xnew"

== system zynqRadioHWSWLTEDetectorAD9361AD9364SL/HDL_LTE/PSS_Detection/Peak_Detection/Local_Search_PSS0/maximum/Delay Reset2/Reset Delay ==
  note: Reset
  u1 : Inport
  R1 : Inport  Port=2
  FixPt Constant : Constant  DisableCoverage=on  Value=0  OutDataTypeStr=fixdt(0,8,0)  SampleTime=simParams.TsRx
  FixPt Logical Operator : Logic  DisableCoverage=on  Operator=OR  AllPortsSameDT=off  OutDataTypeStr=fixdt(0, 8)
  FixPt Unit Delay1 : UnitDelay  DisableCoverage=on  SampleTime=-1  HasFrameUpgradeWarning=off
  FixPt Unit Delay2 : UnitDelay  DisableCoverage=on  InitialCondition=1  SampleTime=-1
  Init : Switch  Criteria=u2 > Threshold  OutDataTypeStr=Inherit: Inherit via back propagation  ZeroCross=off
  Initial Condition : Constant  DisableCoverage=on  Value=0  OutDataTypeStr=Inherit: Inherit via back propagation  SampleTime=simParams.TsRx
  Reset : Switch  Criteria=u2 > Threshold  OutDataTypeStr=Inherit: Inherit via back propagation  ZeroCross=off
  Out1 : Outport
  wires:
  u1/1 -> Reset/3
  FixPt Unit Delay1/1 -> Init/3  "Xold"
  Initial Condition/1 -> Init/1, Reset/1  "Initial Value"
  FixPt Constant/1 -> FixPt Unit Delay2/1
  FixPt Unit Delay2/1 -> FixPt Logical Operator/2
  FixPt Logical Operator/1 -> Init/2
  R1/1 -> FixPt Logical Operator/1, Reset/2
  Init/1 -> Out1/1
  Reset/1 -> FixPt Unit Delay1/1  "Xnew"

== system zynqRadioHWSWLTEDetectorAD9361AD9364SL/HDL_LTE/PSS_Detection/Peak_Detection/Local_Search_PSS1/maximum/Delay Reset/Reset Delay ==
  note: Reset
  u1 : Inport
  R1 : Inport  Port=2
  FixPt Constant : Constant  DisableCoverage=on  Value=0  OutDataTypeStr=fixdt(0,8,0)  SampleTime=simParams.TsRx
  FixPt Logical Operator : Logic  DisableCoverage=on  Operator=OR  AllPortsSameDT=off  OutDataTypeStr=fixdt(0, 8)
  FixPt Unit Delay1 : UnitDelay  DisableCoverage=on  SampleTime=-1  HasFrameUpgradeWarning=off
  FixPt Unit Delay2 : UnitDelay  DisableCoverage=on  InitialCondition=1  SampleTime=-1
  Init : Switch  Criteria=u2 > Threshold  OutDataTypeStr=Inherit: Inherit via back propagation  ZeroCross=off
  Initial Condition : Constant  DisableCoverage=on  Value=0  OutDataTypeStr=Inherit: Inherit via back propagation  SampleTime=simParams.TsRx
  Reset : Switch  Criteria=u2 > Threshold  OutDataTypeStr=Inherit: Inherit via back propagation  ZeroCross=off
  Out1 : Outport
  wires:
  Reset/1 -> FixPt Unit Delay1/1  "Xnew"
  Init/1 -> Out1/1
  R1/1 -> Reset/2, FixPt Logical Operator/1
  FixPt Logical Operator/1 -> Init/2
  FixPt Unit Delay2/1 -> FixPt Logical Operator/2
  FixPt Constant/1 -> FixPt Unit Delay2/1
  Initial Condition/1 -> Reset/1, Init/1  "Initial Value"
  FixPt Unit Delay1/1 -> Init/3  "Xold"
  u1/1 -> Reset/3

== system zynqRadioHWSWLTEDetectorAD9361AD9364SL/HDL_LTE/PSS_Detection/Peak_Detection/Local_Search_PSS1/maximum/Delay Reset2/Reset Delay ==
  note: Reset
  u1 : Inport
  R1 : Inport  Port=2
  FixPt Constant : Constant  DisableCoverage=on  Value=0  OutDataTypeStr=fixdt(0,8,0)  SampleTime=simParams.TsRx
  FixPt Logical Operator : Logic  DisableCoverage=on  Operator=OR  AllPortsSameDT=off  OutDataTypeStr=fixdt(0, 8)
  FixPt Unit Delay1 : UnitDelay  DisableCoverage=on  SampleTime=-1  HasFrameUpgradeWarning=off
  FixPt Unit Delay2 : UnitDelay  DisableCoverage=on  InitialCondition=1  SampleTime=-1
  Init : Switch  Criteria=u2 > Threshold  OutDataTypeStr=Inherit: Inherit via back propagation  ZeroCross=off
  Initial Condition : Constant  DisableCoverage=on  Value=0  OutDataTypeStr=Inherit: Inherit via back propagation  SampleTime=simParams.TsRx
  Reset : Switch  Criteria=u2 > Threshold  OutDataTypeStr=Inherit: Inherit via back propagation  ZeroCross=off
  Out1 : Outport
  wires:
  Reset/1 -> FixPt Unit Delay1/1  "Xnew"
  Init/1 -> Out1/1
  R1/1 -> Reset/2, FixPt Logical Operator/1
  FixPt Logical Operator/1 -> Init/2
  FixPt Unit Delay2/1 -> FixPt Logical Operator/2
  FixPt Constant/1 -> FixPt Unit Delay2/1
  Initial Condition/1 -> Reset/1, Init/1  "Initial Value"
  FixPt Unit Delay1/1 -> Init/3  "Xold"
  u1/1 -> Reset/3

== system zynqRadioHWSWLTEDetectorAD9361AD9364SL/HDL_LTE/PSS_Detection/Peak_Detection/Local_Search_PSS2/maximum/Delay Reset/Reset Delay ==
  note: Reset
  u1 : Inport
  R1 : Inport  Port=2
  FixPt Constant : Constant  DisableCoverage=on  Value=0  OutDataTypeStr=fixdt(0,8,0)  SampleTime=simParams.TsRx
  FixPt Logical Operator : Logic  DisableCoverage=on  Operator=OR  AllPortsSameDT=off  OutDataTypeStr=fixdt(0, 8)
  FixPt Unit Delay1 : UnitDelay  DisableCoverage=on  SampleTime=-1  HasFrameUpgradeWarning=off
  FixPt Unit Delay2 : UnitDelay  DisableCoverage=on  InitialCondition=1  SampleTime=-1
  Init : Switch  Criteria=u2 > Threshold  OutDataTypeStr=Inherit: Inherit via back propagation  ZeroCross=off
  Initial Condition : Constant  DisableCoverage=on  Value=0  OutDataTypeStr=Inherit: Inherit via back propagation  SampleTime=simParams.TsRx
  Reset : Switch  Criteria=u2 > Threshold  OutDataTypeStr=Inherit: Inherit via back propagation  ZeroCross=off
  Out1 : Outport
  wires:
  u1/1 -> Reset/3
  FixPt Unit Delay1/1 -> Init/3  "Xold"
  Initial Condition/1 -> Init/1, Reset/1  "Initial Value"
  FixPt Constant/1 -> FixPt Unit Delay2/1
  FixPt Unit Delay2/1 -> FixPt Logical Operator/2
  FixPt Logical Operator/1 -> Init/2
  R1/1 -> FixPt Logical Operator/1, Reset/2
  Init/1 -> Out1/1
  Reset/1 -> FixPt Unit Delay1/1  "Xnew"

== system zynqRadioHWSWLTEDetectorAD9361AD9364SL/HDL_LTE/PSS_Detection/Peak_Detection/Local_Search_PSS2/maximum/Delay Reset2/Reset Delay ==
  note: Reset
  u1 : Inport
  R1 : Inport  Port=2
  FixPt Constant : Constant  DisableCoverage=on  Value=0  OutDataTypeStr=fixdt(0,8,0)  SampleTime=simParams.TsRx
  FixPt Logical Operator : Logic  DisableCoverage=on  Operator=OR  AllPortsSameDT=off  OutDataTypeStr=fixdt(0, 8)
  FixPt Unit Delay1 : UnitDelay  DisableCoverage=on  SampleTime=-1  HasFrameUpgradeWarning=off
  FixPt Unit Delay2 : UnitDelay  DisableCoverage=on  InitialCondition=1  SampleTime=-1
  Init : Switch  Criteria=u2 > Threshold  OutDataTypeStr=Inherit: Inherit via back propagation  ZeroCross=off
  Initial Condition : Constant  DisableCoverage=on  Value=0  OutDataTypeStr=Inherit: Inherit via back propagation  SampleTime=simParams.TsRx
  Reset : Switch  Criteria=u2 > Threshold  OutDataTypeStr=Inherit: Inherit via back propagation  ZeroCross=off
  Out1 : Outport
  wires:
  u1/1 -> Reset/3
  FixPt Unit Delay1/1 -> Init/3  "Xold"
  Initial Condition/1 -> Init/1, Reset/1  "Initial Value"
  FixPt Constant/1 -> FixPt Unit Delay2/1
  FixPt Unit Delay2/1 -> FixPt Logical Operator/2
  FixPt Logical Operator/1 -> Init/2
  R1/1 -> FixPt Logical Operator/1, Reset/2
  Init/1 -> Out1/1
  Reset/1 -> FixPt Unit Delay1/1  "Xnew"

== matlab function zynqRadioHWSWLTEDetectorAD9361AD9364SL/HDL_LTE/PSS_Detection/Determine_Primary_Cell_ID/PipelinedMax ==
  data: x input; val output; idx output uint16
function [val,idx] = PipelinedMax(x)
    % Returns the maximum value in the vector x. x must be of length 3.
    % This requires two comparisons. To optimized for HDL timing performance,
    % a single register is placed between the two comparisons.
    %#codegen
    
    persistent valReg;    % max value out of 1 and 2
    persistent idxReg;    % zero based index
    
    if isempty(valReg)
        valReg = cast(0,'like',x(1));
        idxReg = uint16(0);
    end
    
    % second comparison, reads registers before they are written to
    if valReg > x(3)
        val = valReg;
        idx = idxReg;
    else
        val = x(3);
        idx = uint16(2);
    end
    
    % first comparison, writes to registers
    if x(1) > x(2)
        valReg(:) = x(1);
        idxReg(:) = uint16(0);
    else
        valReg(:) = x(2);
        idxReg(:) = uint16(1);
    end
    
end

== matlab function zynqRadioHWSWLTEDetectorAD9361AD9364SL/Decode and Print/PrintCellID ==
  data: u input
function printCellID(u)
%#codegen

% Create empty 2-element array of zeros
b = fi(complex(zeros(2,1), zeros(2,1)),1,16,0);

% Get 2 fields from array (samples are interleaved, and upsampled 32x, so
% get last sample, and the 33rd last...
b(1) = fi(u(end),1,16,0);
b(2) = fi(u(end-33),1,16,0);

% Determine which is freq estimate using flag bit
if bitget(imag(b(1)),16) == 1
    freqEst = double(real(b(1)));
    pCellID = int16(bitsliceget(imag(b(2)),2,1));
    sCellID = int16(bitsliceget(imag(b(2)),10,3));
    CellID = int16(bitsliceget(real(b(2)),9,1));
else
    freqEst = double(real(b(2)));
    pCellID = int16(bitsliceget(imag(b(1)),2,1));
    sCellID = int16(bitsliceget(imag(b(1)),10,3));
    CellID = int16(bitsliceget(real(b(1)),9,1));
end

% Scale freq estimate back to double, and multiply by carrier spacing of 15
% kHz
freqEst = (freqEst/2^9)*15000;

% Print out to console
fprintf('-------------------------------\n');
fprintf(['Detected Cell ID: %i\n        ' ...
         'PCell ID: %i\n        ' ...
         'SCell ID: %i\n' ...
         '-------------------------------\n' ...
         'Freq Est:         %0.3f Hz\n'], ...
         CellID, pCellID, sCellID, freqEst);
fprintf('-------------------------------\n');
